simulink model "forward_speed_model_ulin"  (R2017b)
settings: Solver=ode45  StartTime=tstart  StopTime=tstop  RelTol=1e-3
values from neighbouring files (symbols this model uses):
  k = lsqcurvefit(F, k0, t, u,[600 0.2 0.09],[1150 0.6  0.13],OPT)    [analyse_dynamics_v3.m]    (also in analysis_dynamics.m = lsqcurvefit(F3,k0,t,u,lb,ub,options))
  tau_1 = n_c    [sim_forward_speed_mass_damp_model.m]    (also in sim_forward_speed_model_ulin.m)
settings Model: Creator=EllaLovise  LastModifiedBy=Alexandra

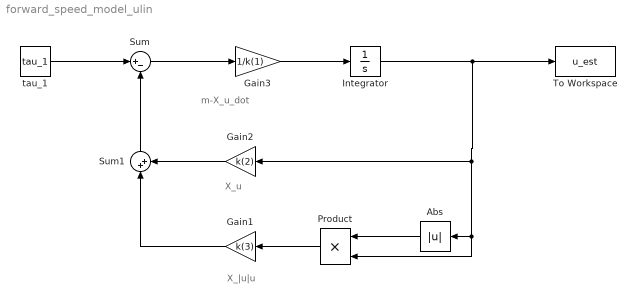
== system forward_speed_model_ulin ==
  note: X_|u|u
  note: X_u
  note: m-X_u_dot
  Abs : Abs
  Gain1 : Gain  Gain=k(3)
  Gain2 : Gain  Gain=k(2)
  Gain3 : Gain  Gain=1/k(1)
  Integrator : Integrator  InitialCondition=6.63
  Product : Product
  Sum : Sum  Inputs=|+-
  Sum1 : Sum  Inputs=|++
  To Workspace : ToWorkspace  VariableName=u_est  SampleTime=100
  tau_1 : Constant  Value=tau_1
  wires:
  tau_1/1 -> Sum/1
  Product/1 -> Gain1/1
  Integrator/1 -> To Workspace/1, Product/2, Abs/1, Gain2/1
  Abs/1 -> Product/1
  Gain1/1 -> Sum1/1
  Sum1/1 -> Sum/2
  Gain2/1 -> Sum1/2
  Gain3/1 -> Integrator/1
  Sum/1 -> Gain3/1
